simulink model "ZiglerNichols_model"  (R2017b)
settings: Solver=FixedStepAuto  StartTime=0.0  StopTime=10.0  FixedStep=0.05  RelTol=1e-3
values from neighbouring files (symbols this model uses):
  G_den = [ 1 6 11 6 ]    [ZieglerNichols_script.m]
  G_num = [5]    [ZieglerNichols_script.m]
settings Model: Creator=Admin  LastModifiedBy=Admin

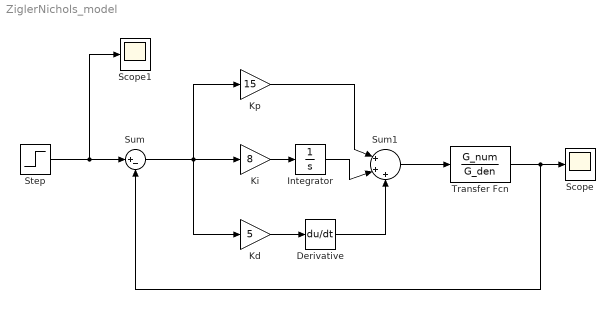
== system ZiglerNichols_model ==
  Derivative : Derivative
  Integrator : Integrator
  "Kd " : Gain  Gain=5
  "Ki " : Gain  Gain=8
  "Kp " : Gain  Gain=15
  Scope : Scope
  Scope1 : Scope
  Step : Step  SampleTime=0
  Sum : Sum  Inputs=|+-
  Sum1 : Sum  Inputs=|+++
  Transfer Fcn : TransferFcn  Numerator=G_num  Denominator=G_den
  wires:
  "Kp "/1 -> Sum1/1
  Sum1/1 -> Transfer Fcn/1
  Sum/1 -> "Kd "/1, "Ki "/1, "Kp "/1
  Step/1 -> Scope1/1, Sum/1
  "Ki "/1 -> Integrator/1
  Integrator/1 -> Sum1/2
  "Kd "/1 -> Derivative/1
  Derivative/1 -> Sum1/3
  Transfer Fcn/1 -> Sum/2, Scope/1
